simulink model "eee_316_stepper_driver"  (R2020a)
settings: Solver=VariableStepAuto  StartTime=0.0  StopTime=inf  FixedStep=0.00001  MaxStep=0.0001  RelTol=10
libraries: fl_lib x39, nesl_utility x11, ee_lib x5, simulink_extras x1
settings Model: Creator=Sadat  LastModifiedBy=User
settings SolverCC: MaxConsecutiveMinStep=10
settings DataIOCC: ReturnWorkspaceOutputs=off
settings DebuggingCC: ArithmeticOperatorsInVariantConditions=warning
settings SFSimCC: CustomCodeUndefinedFunction=UseInterfaceOnly

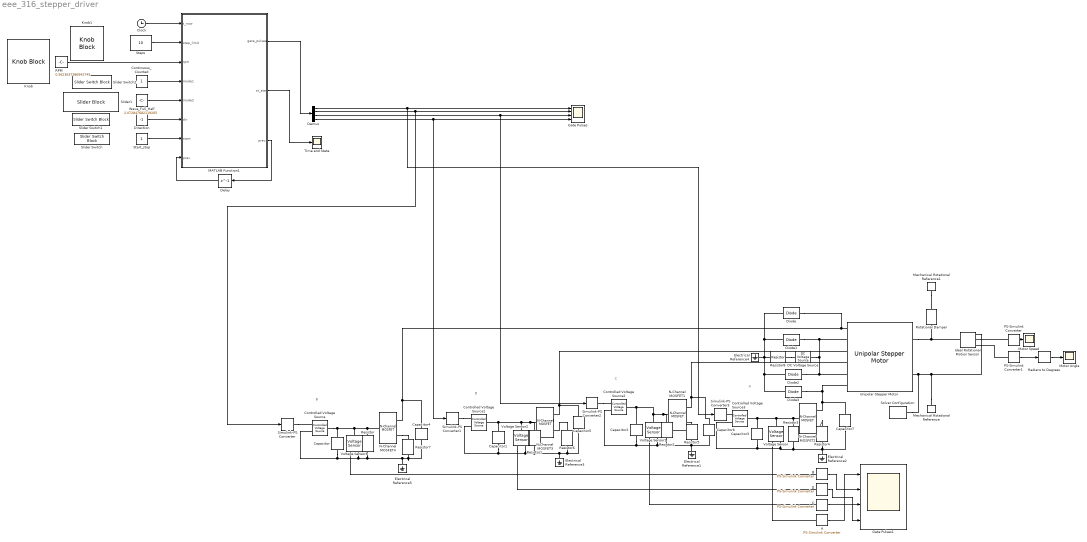
== system eee_316_stepper_driver ==
  note: D
  note: B
  note: A
  note: C
  A : nesl_utility/PS-Simulink Converter  PhysicalDomain=network_engine_domain  SubClassName=ps_output  LeftPortType=input  RightPortType=output  PseudoPeriodic=off  Frequencies=[]  Unit=1  AffineConversion=off
  B : nesl_utility/PS-Simulink Converter  PhysicalDomain=network_engine_domain  SubClassName=ps_output  LeftPortType=input  RightPortType=output  PseudoPeriodic=off  Frequencies=[]  Unit=1  AffineConversion=off
  C : nesl_utility/PS-Simulink Converter  PhysicalDomain=network_engine_domain  SubClassName=ps_output  LeftPortType=input  RightPortType=output  PseudoPeriodic=off  Frequencies=[]  Unit=1  AffineConversion=off
  Capacitor{,1..3} (4 alike) : fl_lib/Electrical/Electrical Elements/Capacitor  c=0.1 F  r=1e-6 Ohm  g=0 1/Ohm  i_specify=off  i_priority=None  i=0 A  i_nominal_specify=off  i_nominal_unit=A  i_nominal_value=1  v_specify=off  v_priority=None  v=0 V  v_nominal_specify=off  v_nominal_unit=V  v_nominal_value=1  vc_specify=off  vc_priority=High  vc=0 V  vc_nominal_specify=off  vc_nominal_unit=V  vc_nominal_value=1
  Capacitor{4..7} (4 alike) : fl_lib/Electrical/Electrical Elements/Capacitor  c=0.1 mF  r=1e-6 Ohm  g=0 1/Ohm  i_specify=off  i_priority=None  i=0 A  i_nominal_specify=off  i_nominal_unit=A  i_nominal_value=1  v_specify=off  v_priority=None  v=0 V  v_nominal_specify=off  v_nominal_unit=V  v_nominal_value=1  vc_specify=off  vc_priority=High  vc=0 V  vc_nominal_specify=off  vc_nominal_unit=V  vc_nominal_value=1
  Clock : Clock
  Continuous_Counted : Constant
  Controlled Voltage Source{,1..3} (4 alike) : fl_lib/Electrical/Electrical Sources/Controlled Voltage Source
  D : nesl_utility/PS-Simulink Converter  PhysicalDomain=network_engine_domain  SubClassName=ps_output  LeftPortType=input  RightPortType=output  PseudoPeriodic=off  Frequencies=[]  Unit=1  AffineConversion=off
  DC Voltage Source : fl_lib/Electrical/Electrical Sources/DC Voltage Source  v0=12 V
  Delay : Delay  DelayLength=1  InitialCondition=[0 1 0 0 0 0 0]
  Demux : Demux
  Diode{,1..3} (4 alike) : fl_lib/Electrical/Electrical Elements/Diode  Vf=0.6 V  Ron=0.3 Ohm  Goff=1e-8 1/Ohm  i_specify=off  i_priority=None  i=0 A  i_nominal_specify=off  i_nominal_unit=A  i_nominal_value=1  v_specify=off  v_priority=None  v=0 V  v_nominal_specify=off  v_nominal_unit=V  v_nominal_value=1
  "Direction " : Constant  Value=-1
  Electrical Reference{1..5} (5 alike) : fl_lib/Electrical/Electrical Elements/Electrical Reference
  Gate Pulses : Scope  NumInputPorts=4
  Gate Pulses1 : Scope  NumInputPorts=4
  Ideal Rotational Motion Sensor : fl_lib/Mechanical/Mechanical Sensors/Ideal Rotational Motion Sensor  wrap_angle=simscape.enum.onoff.off  offset=0 rad
  Knob : KnobBlock  ScaleMin=0.1  ScaleMax=20  ScaleType=Log
  Knob1 : KnobBlock  ScaleMax=200
  MATLAB Function1 : MATLAB Function  TreatAsAtomicUnit=on
  Mechanical Rotational Reference : fl_lib/Mechanical/Rotational Elements/Mechanical Rotational Reference
  Mechanical Rotational Reference1 : fl_lib/Mechanical/Rotational Elements/Mechanical Rotational Reference
  Motor Angle : Scope
  Motor Speed : Scope
  N-Channel MOSFET{1..4} (4 alike) : ee_lib/Semiconductors & Converters/N-Channel MOSFET  paramTerminal=ee.enum.mosfet.numberOfTerminals.three  parameterization=ee.enum.parameterization.datasheet  prmDatasheet=ee.enum.temperatureParameterization.none  prmEquCoeff=ee.enum.temperatureParameterization.none  Beta=5 A/V^2  Rds=0.1 Ohm  Id=6 A  Vgs=10 V  Vth=3 V  Vth0=1.7 V  lam=0 1/V  gamma_vth=0.5 V^0.50000  phib=0.5 V  Vth1=1.9071 V  Vbs1=-1 V  Vth2=2.066 V  Vbs2=-2 V  Tmeas=25 degC  RS=1e-4 Ohm  RD=0.01 Ohm  RB=0.001 Ohm  C_param=ee.enum.mosfet.capacitanceParam.fixedciss  C_GS=270 pF  C_GD=80 pF  C_DS=0 pF  C_iss=350 pF  C_rss=80 pF  C_oss=0 pF  charge_linearity_param=ee.enum.mosfet.cgdLinearity.constant  C_OX=200 pF  V_C_OX=-0.5 V  C_iss_vec=[ 720 700 590 470 390 310 ] pF  C_rss_vec=[ 450 400 300 190 95 55 ] pF  C_oss_vec=[ 900 810 690 420 270 170 ] pF  C_GS_vec=[ 270 300 290 280 295 255 ] pF  C_GD_vec=[ 450 400 300 190 95 55 ] pF  C_DS_vec=[ 450 410 390 230 175 115 ] pF  C_Vds_vec=[ 0.1 0.3 1 3 10 30 ] V  V_GS_for_cap_data=0 V  charge_linearity_param_vgb=ee.enum.mosfet.cgbLinearity.instantly  IsDiode=0 A  Vbi=0.6 V  n=1  Cj0Diode=0 pF  TT=50e-9 s  dVth_dT=-6 mV/K  dVth0_dT=-6 mV/K  Rds_T2=0.037 Ohm  Tmeas2=125 degC  BEXDatasheet=-1.5  BEXEquCoeff=-1.5  etaisDatasheet=3  etaisEquCoeff=3  TdeviceDatasheet=25 degC  TdeviceEquCoeff=25 degC  thermal_network_parameterization=ee.enum.thermalNetworkTopology.cauer  Rth=[0, 10] K/W  Rth_Foster=[4, 6] K/W  thermal_mass_parameterization=ee.enum.thermalNetwork.timeconstant  thermal_mass=[0, 1] J/K  thermal_mass_Foster=[1.5, 3] J/K  thermal_time_constant=[0, 10] s  thermal_time_constant_Foster=[6, 18] s  thermal_mass_initial_temperatures=[25, 25] degC  betaref=18 A/V^2  Vfbref=-1.1 V  gamma=3.5 V^0.50000  phib2ref=1 V  thesatref=0.4 1/V  alpha=0  Vp=5e-2 V  thesrref=0 1/V  m=8  Tref=25 degC  Cox=1500 pF  Cgso=100 pF  Cgdo=14 pF  Rsref=2e-3 Ohm  Rdref=0.17 Ohm  Rgref=8.4 Ohm  Rbref=2e-3 Ohm  Isref=5.2e-13 A  Cj0=480 pF  Tprm=1  etabet=1.3  Stvfb=5e-4 V/K  Stphib=-8.5e-4 V/K  etasat=1.04  etasr=0.65  etar=0.95  etais=3  Tsim=25 degC  T0=[25, 25] degC
  PS-Simulink Converter : nesl_utility/PS-Simulink Converter  PhysicalDomain=network_engine_domain  SubClassName=ps_output  LeftPortType=input  RightPortType=output  PseudoPeriodic=off  Frequencies=[]  Unit=1  AffineConversion=off
  PS-Simulink Converter1 : nesl_utility/PS-Simulink Converter  PhysicalDomain=network_engine_domain  SubClassName=ps_output  LeftPortType=input  RightPortType=output  PseudoPeriodic=off  Frequencies=[]  Unit=rad  AffineConversion=off
  RPM : Constant  Value=0.5623637386942745
  Radians to Degrees : simulink_extras/Transformations/Radians to Degrees
  Resistor{,1..8} (9 alike) : fl_lib/Electrical/Electrical Elements/Resistor  R=1 Ohm  i_specify=off  i_priority=None  i=0 A  i_nominal_specify=off  i_nominal_unit=A  i_nominal_value=1  v_specify=off  v_priority=None  v=0 V  v_nominal_specify=off  v_nominal_unit=V  v_nominal_value=1
  Rotational Damper : fl_lib/Mechanical/Rotational Elements/Rotational Damper  D=0.5 N*m/(rad/s)  w_specify=off  w_priority=None  w=0 rad/s  w_nominal_specify=off  w_nominal_unit=rad/s  w_nominal_value=1  t_specify=off  t_priority=None  t=0 N*m  t_nominal_specify=off  t_nominal_unit=N*m  t_nominal_value=1
  Simulink-PS Converter{,1..3} (4 alike) : nesl_utility/Simulink-PS Converter  PhysicalDomain=network_engine_domain  SubClassName=ps_input  LeftPortType=input  RightPortType=output  PseudoPeriodic=off  Frequencies=[]  NoiseDistribution=none  NoiseParameters=[]  Unit=1  AffineConversion=off  FilteringAndDerivatives=provide  SimscapeFilterOrder=1  InputFilterTimeConstant=0.001  UdotUserProvided=0
  Slider Switch : SliderSwitchBlock
      settings: Values={{'Stop', 'Start'}, [0 1]}
  Slider Switch1 : SliderSwitchBlock
      settings: Values={{'Backward', 'Forward'}, [-1 1]}
  Slider Switch2 : SliderSwitchBlock
      settings: Values={{'Continuous', 'Counted'}, [1 2]}
  Slider1 : SliderBlock  ScaleMin=1  ScaleMax=3  TickInterval=1
  Solver Configuration : nesl_utility/Solver Configuration  PhysicalDomain=network_engine_domain  SubClassName=solver  LeftPortType=input  RightPortType=generic  Tones=[]  Harmonics=[]  SimulateNoise=off  Profile=off  UseLocalSampling=off  EnableSwitchedLinearOptims=on  FrequencyDomain=off  UseCCode=off  RelTol=0.001  AbsTol=1e-06  MinStep=1e-09  ToWorkspace=off  RevertToSquareIcSolve=off  NumHomotopyIterations=100  PhasorMode=off  PhasorModeNumHarmonics=1  DoDC=off  ResidualTolerance=1e-09  UseLocalSolver=off  LocalSolverChoice=NE_BACKWARD_EULER_ADVANCER  LocalSolverSampleTime=0.001  DoFixedCost=off  MaxNonlinIter=3  MaxModeIter=2  LinearAlgebra=Sparse  EquationFormulation=NE_TIME_EF  DelaysMemoryBudget=1024  AutomaticFiltering=on  FilteringTimeConstant=0.001  PartitionStorageMethod=AS_NEEDED  PartitionMemoryBudget=1024  PartitionMethod=FAST
  "Start_stop " : Constant
  Steps : Constant  Value=10
  Time and State : Scope
  Unipolar Stepper Motor : ee_lib/Electromechanical/Reluctance & Stepper/Unipolar Stepper Motor  step_or_av=1  w_vec=[0, 1000, 3000] rpm  T_vec=[2, 2, 1] N*m  assert_if_slipping=0  J_total=1e-4 kg*m^2  max_step_rate=10 Hz  Ra=0.75 Ohm  La=1.5e-3 H  Km=1.1 N*m/A  Td=0 N*m  Rm=99999 Ohm  Step=1.8 deg  J=4.5e-5 kg*m^2  B=8.0e-4 N*m/(rad/s)  speed0=0 rpm  theta0=0 deg  alpha=3.93e-3 1/K  Tmeas=25 degC  T_vec2=[1.7, 1.7, .85] N*m  Tmeas2=125 degC  half_stepping=0  thermal_mass=100 J/K  initial_temperatures=[25, 25, 25, 25] degC  rotor_thermal_mass=50 J/K  rotor_initial_temperature=25 degC  Rm_percent_rotor=90
      settings: SourceProductBaseCode=PS  InternalSimscapePortConfiguration="{\"Bottom\":[],\"Left\":[{\"id\":\"pA\",\"label\":\"A+\",\"type\":\"foundation.electrical.electrical\"},{\"id\":\"cA\",\"label\":\"A0\",\"type\":\"foundation.electrical.electrical\"},{\"id\":\"nA\",\"label\":\"A-\",\"type\":\"foundation.electrical.electrical\"},{\"id\":\"pB\",\"label\":\"B+\",\"type\":\"foundation.electrical.electrical\"},{\"id\":\"cB\",\"label\":\"B0\",\"type\":\"foundation.electrical.electrical\"},{\"id\":\"nB\",\"label\":\"B-\",\"type\":\"foundation.electrical.electrical\"}],\"Right\":[{\"id\":\"R\",\"label\":\"R\",\"type\":\"foundation.mechanical.rotational.rotational\"},{\"id\":\"C\",\"label\":\"C\",\"type\":\"foundation.mechanical.rotational.rotational\"}],\"Top\":[]}"
  Voltage Sensor{,1..3} (4 alike) : fl_lib/Electrical/Electrical Sensors/Voltage Sensor
  Wave_Full_Half : Constant  Value=2.072847682119205
  wires:
  MATLAB Function1/1(gate_pulses) -> Demux/1
  Demux/2 -> Simulink-PS Converter/1, Gate Pulses/2
  Demux/1 -> Simulink-PS Converter3/1, Gate Pulses/1
  Demux/4 -> Simulink-PS Converter1/1, Gate Pulses/4
  Demux/3 -> Simulink-PS Converter2/1, Gate Pulses/3
  Radians to Degrees/1 -> Motor Angle/1
  PS-Simulink Converter/1 -> Motor Speed/1
  PS-Simulink Converter1/1 -> Radians to Degrees/1
  MATLAB Function1/3(prev) -> Delay/1
  Delay/1 -> MATLAB Function1/8("prev ")
  Wave_Full_Half/1 -> MATLAB Function1/5(mode2)
  "Direction "/1 -> MATLAB Function1/6(dir)
  "Start_stop "/1 -> MATLAB Function1/7(start)
  Continuous_Counted/1 -> MATLAB Function1/4(mode1)
  Steps/1 -> MATLAB Function1/2(step_limit)
  RPM/1 -> MATLAB Function1/3(rpm)
  Clock/1 -> MATLAB Function1/1(t_now)
  MATLAB Function1/2(st_ate) -> Time and State/1
  A/1 -> Gate Pulses1/1
  C/1 -> Gate Pulses1/3
  B/1 -> Gate Pulses1/2
  D/1 -> Gate Pulses1/4
  connections:
  Mechanical Rotational Reference/LConn1 -- Unipolar Stepper Motor/RConn2 -- Solver Configuration/RConn1 -- Ideal Rotational Motion Sensor/RConn1
  Capacitor/RConn1 -- Controlled Voltage Source/RConn2 -- Voltage Sensor3/RConn2 -- Resistor/RConn1 -- Resistor7/RConn1 -- Capacitor4/RConn1 -- Electrical Reference5/LConn1
  Diode1/RConn1 -- Unipolar Stepper Motor/LConn2 -- DC Voltage Source/LConn1 -- Diode2/RConn1 -- Unipolar Stepper Motor/LConn5
  Resistor3/LConn1 -- N-Channel MOSFET2/LConn1 -- Voltage Sensor/LConn1 -- Capacitor3/LConn1 -- Controlled Voltage Source3/LConn1
  Capacitor3/RConn1 -- Controlled Voltage Source3/RConn2 -- Voltage Sensor/RConn2 -- Resistor3/RConn1 -- Resistor4/RConn1 -- Capacitor7/RConn1 -- Electrical Reference2/LConn1
  Voltage Sensor2/RConn2 -- Resistor6/RConn1 -- Capacitor5/RConn1 -- Electrical Reference3/LConn1 -- Resistor1/RConn1 -- Capacitor1/RConn1 -- Controlled Voltage Source1/RConn2
  N-Channel MOSFET3/RConn1 -- Unipolar Stepper Motor/LConn3 -- Capacitor5/LConn1
  Rotational Damper/LConn1 -- Unipolar Stepper Motor/RConn1 -- Ideal Rotational Motion Sensor/LConn1
  Voltage Sensor1/RConn2 -- Controlled Voltage Source2/RConn2 -- Capacitor2/RConn1 -- Capacitor6/RConn1 -- Resistor5/RConn1 -- Electrical Reference1/LConn1 -- Resistor2/RConn1
  N-Channel MOSFET1/LConn1 -- Voltage Sensor1/LConn1 -- Capacitor2/LConn1 -- Controlled Voltage Source2/LConn1 -- Resistor2/LConn1
  N-Channel MOSFET3/LConn1 -- Resistor1/LConn1 -- Voltage Sensor2/LConn1 -- Controlled Voltage Source1/LConn1 -- Capacitor1/LConn1
  N-Channel MOSFET1/RConn1 -- Capacitor6/LConn1 -- Unipolar Stepper Motor/LConn4
  N-Channel MOSFET4/RConn1 -- Capacitor4/LConn1 -- Diode/RConn1 -- Unipolar Stepper Motor/LConn1
  Controlled Voltage Source/LConn1 -- Capacitor/LConn1 -- N-Channel MOSFET4/LConn1 -- Resistor/LConn1 -- Voltage Sensor3/LConn1
  N-Channel MOSFET2/RConn1 -- Unipolar Stepper Motor/LConn6 -- Diode3/RConn1 -- Capacitor7/LConn1
  Voltage Sensor1/RConn1 -- C/LConn1
  PS-Simulink Converter/LConn1 -- Ideal Rotational Motion Sensor/RConn2
  PS-Simulink Converter1/LConn1 -- Ideal Rotational Motion Sensor/RConn3
  Mechanical Rotational Reference1/LConn1 -- Rotational Damper/RConn1
  Voltage Sensor/RConn1 -- A/LConn1
  Simulink-PS Converter3/RConn1 -- Controlled Voltage Source3/RConn1
  Voltage Sensor2/RConn1 -- D/LConn1
  Simulink-PS Converter/RConn1 -- Controlled Voltage Source/RConn1
  Simulink-PS Converter2/RConn1 -- Controlled Voltage Source2/RConn1
  Simulink-PS Converter1/RConn1 -- Controlled Voltage Source1/RConn1
  Voltage Sensor3/RConn1 -- B/LConn1
  Resistor4/LConn1 -- N-Channel MOSFET2/RConn2
  N-Channel MOSFET1/RConn2 -- Resistor5/LConn1
  N-Channel MOSFET3/RConn2 -- Resistor6/LConn1
  N-Channel MOSFET4/RConn2 -- Resistor7/LConn1
  Resistor8/RConn1 -- Diode1/LConn1 -- Diode/LConn1 -- Diode2/LConn1 -- Diode3/LConn1 -- Electrical Reference4/LConn1
  Resistor8/LConn1 -- DC Voltage Source/RConn1

== matlab function eee_316_stepper_driver/MATLAB Function1 ==
  data: gate_pulses output; t_now input; st_ate output; step_limit input; rpm input; mode1 input; mode2 input; dir input; start input; prev output; prev input
function [gate_pulses,st_ate,prev] = stepper_driver(t_now, step_limit, rpm, mode1, mode2, dir, start, prev)

t_prev=prev(1);
state=prev(2);
mode1_prev=prev(3);
mode2_prev=prev(4);
dir_prev=prev(5);
start_prev=prev(6);
steps=prev(7);

step_limit = round(step_limit);
% mode1 = 2;  % 1=continuous, 2=numbered
mode2 = round(mode2);  % 1=wave drive, 2=full step, 3=half step
T = 60/rpm;
step_size=T/(200 + 200*(mode2==3));
% dir   = 1;  % -1 = backward, 1 = forward

%Transition
if start~=start_prev || mode2~=mode2_prev || dir~=dir_prev %|| mode1~=mode1_prev
    %Transition took place
    start_prev=start;
    mode1_prev=mode1;
    mode2_prev=mode2;
    dir_prev=dir;
    %RESET Steps
    steps=0;
end

st_mat= [1 0 0 0;
         1 1 0 0;
         0 1 0 0;
         0 1 1 0;
         0 0 1 0;
         0 0 1 1;
         0 0 0 1;
         1 0 0 1;];

if (t_now-t_prev)>=step_size %Counting Time
    t_prev=t_prev+step_size;
    
    if start==1 && (steps<step_limit || mode1 == 1) %Running Motor
        steps=steps+1;
        
        %Wave Drive
        if mode2==1 %continuous
            if mod(state,2)==0
                state=mod(state+dir,8);
            else
                state=mod(state + dir*2,8);
            end
        end
        
        %Full Step
        if mode2==2 %continuous
            if mod(state,2)==1
                state=state+dir;
            else
                state=mod(state + 2*dir,8);
            end
            
            if state==0
                state=8;
            end
        end
        
        %Half step
        if mode2==3 %continuous
            state = mod(state+dir,8);
            
            if state==0
                state=8;
            end
        end
    end
end

gate_pulses=5*st_mat(state, :);
st_ate=state;
prev=[t_prev; state; mode1_prev; mode2_prev; dir_prev; start_prev; steps];
end
